simulink model "blockDiagramTask7"  (R2025a)
settings: Solver=VariableStepAuto  StartTime=0.0  StopTime=3.6  RelTol=1e-3
InitFcn:
  | run motor_specs.m
model workspace: external: MATLAB File motor_specs.m (data not in the file)
values from neighbouring files (symbols this model uses):
  A6 = [ 0, 0, 1, 0 ... (first row only)    [ssAndTF.m]
  B6 = [0, 0, K_M/(J_gm*R), 0]'    [ssAndTF.m]
  b_m = C_V / rpm_to_rs    (= 1.05042262441e-05)    [motor_specs.m]
  C6 = eye(4)    [ssAndTF.m]
  J = 6.3E-6    (= 6.3e-06)    [motor_specs.m]
  K_E = 0.006741 / rpm_to_rs    (= 0.0643718082829)    [motor_specs.m]
  K_M = 0.0644    [motor_specs.m]
  R = 3.23    [motor_specs.m]
  U_N = 36    [motor_specs.m]
undefined symbols (not defined in the file or in its folder): sigbuilder_block
libraries: fl_lib x4, nesl_utility x3, ee_lib x1, slpidlib x1
settings Model: Creator=josef  LastModifiedBy=josef

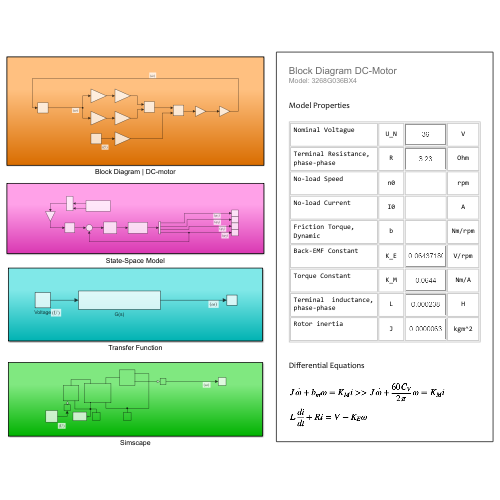
[thumbnail: Simulink's stored preview of the top-level diagram]
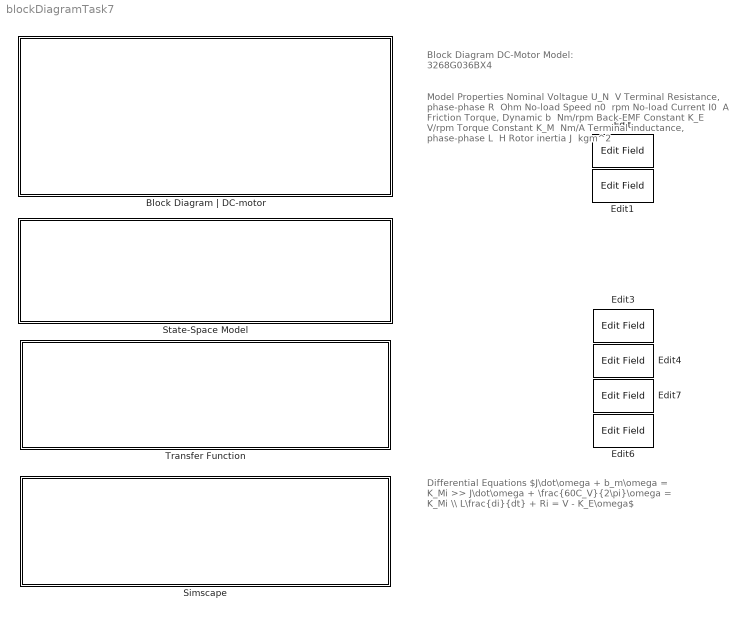
== system blockDiagramTask7 ==
  note: Differential Equations
      |
      | $J\dot\omega + b_m\omega = K_Mi >> J\dot\omega + \frac{60C_V}{2\pi}\omega = K_Mi \\ L\frac{di}{dt} + Ri = V - K_E\omega$
  note: Model Properties
      |
      | Nominal Voltague
      |
      | U_N
      | ​
      | V
      |
      | Terminal Resistance,
      | phase-phase
      | R
      | ​
      | Ohm
      |
      | No-load Speed
      |
      | n0
      | ​
      | rpm
      |
      | No-load Current
      |
      | I0
      | ​
      | A
      |
      | Friction Torque,
      | Dynamic
      | b
      | ​
      | Nm/rpm
      |
      | Back-EMF Constant
      |
      | K_E
      | ​
      | V/rpm
      |
      | Torque Constant
      |
      | K_M
      | ​
      | Nm/A
      |
      | Terminal inductance,
      | phase-phase
      | L
      | ​
      | H
      |
      | Rotor inertia
      |
      | J
      | ​
      | kgm^2
  note: Block Diagram DC-Motor
      | Model: 3268G036BX4
  Block Diagram | DC-motor : Subsystem
  Edit{,1,3..4,6..7} (6 alike) : EditField  LabelPosition=Hide  ShowInitialText=on  Alignment=Center  Opacity=0
  Simscape : Subsystem
  State-Space Model : Subsystem
  Transfer Function : Subsystem

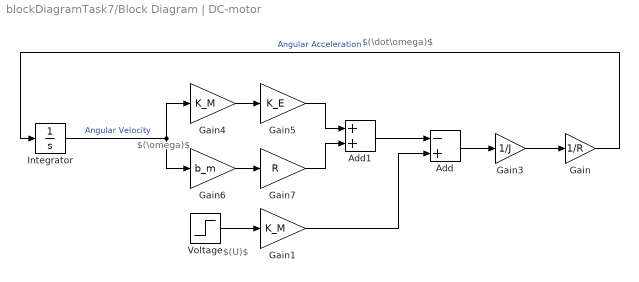
== system blockDiagramTask7/Block Diagram | DC-motor ==
  note: $(\omega)$
  note: $(\dot\omega)$
  note: $(U)$
  Add : Sum  Inputs=-+
  Add1 : Sum
  Gain : Gain  Gain=1/R
  Gain1 : Gain  Gain=K_M
  Gain3 : Gain  Gain=1/J
  Gain4 : Gain  Gain=K_M
  Gain5 : Gain  Gain=K_E
  Gain6 : Gain  Gain=b_m
  Gain7 : Gain  Gain=R
  Integrator : Integrator
  Voltage : Step  Time=0  After=U_N  SampleTime=0
  wires:
  Add1/1 -> Add/1
  Gain4/1 -> Gain5/1
  Gain1/1 -> Add/2
  Gain3/1 -> Gain/1
  Gain5/1 -> Add1/1
  Integrator/1 -> Gain6/1, Gain4/1  "Angular Velocity"
  Gain6/1 -> Gain7/1
  Voltage/1 -> Gain1/1
  Gain/1 -> Integrator/1  "Angular Acceleration"
  Gain7/1 -> Add1/2
  Add/1 -> Gain3/1

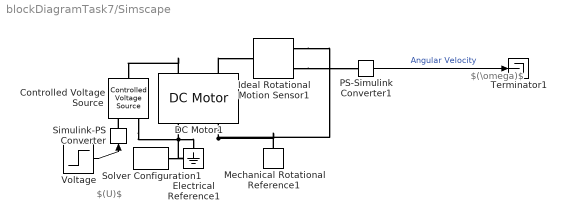
== system blockDiagramTask7/Simscape ==
  note: $(\omega)$
  note: $(U)$
  Controlled Voltage Source : fl_lib/Electrical/Electrical Sources/Controlled Voltage Source
  DC Motor1 : ee_lib/Electromechanical/Brushed Motors/DC Motor  field_option=ee.enum.field_option.pm  Rf=100 Ohm  Lf=1 H  Laf=0.15 H  If0=0 A  parameterization=ee.enum.dcparam_option.circuit_param  Ra=R Ohm  La=0 H  emf_or_torque=ee.enum.emf_or_torque.kv  Kv=K_E V*s/rad  Ki=6.876e-4 N*m/A  T_stall=0.24e-3 N*m  w_max=19100 rpm  w_rated=15000 rpm  P_rated=0.08 W  V_rated=1.5 V  lam_param=ee.enum.lam_param.damping  i_noload=0 A  V_i_noload=1.5 V  J=J kg*m^2  lam=b_m N*m*s/rad  speed0=0 rpm  alpha=3.93e-3 1/K  Tmeas=25 degC  thermal_mass=100 J/K  initial_temperature=25 degC
  Electrical Reference1 : fl_lib/Electrical/Electrical Elements/Electrical Reference
  Ideal Rotational Motion Sensor1 : fl_lib/Mechanical/Mechanical Sensors/Ideal Rotational Motion Sensor  reference=foundation.enum.MeasurementReference.difference  acceleration_port=false  velocity_port=true  position_port=false  wrap_angle=false  offset=0 rad
      settings: InternalSimscapePortConfiguration="{\"Bottom\":[],\"Left\":[{\"id\":\"R\",\"label\":\"R\",\"type\":\"foundation.mechanical.rotational.rotational\"}],\"Right\":[{\"id\":\"C\",\"label\":\"C\",\"type\":\"foundation.mechanical.rotational.rotational\"},{\"id\":\"W\",\"label\":\"W\",\"type\":\"output\"}],\"Top\":[]}"
  Mechanical Rotational Reference1 : fl_lib/Mechanical/Rotational Elements/Mechanical Rotational Reference
  PS-Simulink Converter1 : nesl_utility/PS-Simulink Converter  PhysicalDomain=network_engine_domain  SubClassName=ps_output  LeftPortType=input  RightPortType=output  PseudoPeriodic=off  Frequencies=[]  VectorFormat=inherit  Unit=inherit  AffineConversion=off
  Simulink-PS Converter : nesl_utility/Simulink-PS Converter  PhysicalDomain=network_engine_domain  SubClassName=ps_input  LeftPortType=input  RightPortType=output  PseudoPeriodic=off  Frequencies=[]  NoiseDistribution=none  NoiseParameters=[]  Unit=1  AffineConversion=off  FilteringAndDerivatives=provide  SimscapeFilterOrder=1  InputFilterTimeConstant=0.001  UdotUserProvided=0
  Solver Configuration1 : nesl_utility/Solver Configuration  PhysicalDomain=network_engine_domain  SubClassName=solver  LeftPortType=input  RightPortType=generic  Tones=[]  Harmonics=[]  SimulateNoise=off  Profile=off  UseLocalSampling=off  EnableSwitchedLinearOptims=on  FrequencyDomain=off  UseCCode=off  RelTol=0.001  AbsTol=0.001  MinStep=1e-09  ToWorkspace=off  RevertToSquareIcSolve=off  NumHomotopyIterations=100  PhasorMode=off  PhasorModeNumHarmonics=1  ConsistencySolver=NEWTON_XTOL_AFTER_FTOL  IndexReductionMethod=DerivativeReplacement  DoDC=off  ResidualTolerance=1e-09  ConsistencyTolSource=GLOBAL  ConsistencyAbsTol=0.001  ConsistencyRelTol=0.001  ConsistencyTolFactor=0.001  UseLocalSolver=off  LocalSolverChoice=NE_BACKWARD_EULER_ADVANCER  ResolveIndetEquations=on  FunctionEvalNumThread=1  LocalSolverSampleTime=0.001  DoFixedCost=off  MaxNonlinIter=3  MaxModeIter=2  ComputeImpulses=off  ImpulseIterations=2  LinearAlgebra=auto  LinearAlgebraNumThread=0  EquationFormulation=NE_TIME_EF  DelaysMemoryBudget=1024  AutomaticFiltering=on  FilteringTimeConstant=0.001  PartitionStorageMethod=AS_NEEDED  PartitionMemoryBudget=1024  PartitionMethod=ROBUST  MultibodyUseLocalSolver=off  MultibodyLocalSolverChoice=ODE1  MultibodyLocalSolverSampleTime=0.001
  Terminator1 : Terminator
  Voltage : Step  Time=0.1  After=U_N  SampleTime=0
  wires:
  PS-Simulink Converter1/1 -> Terminator1/1  "Angular Velocity"
  Voltage/1 -> Simulink-PS Converter/1
  connections:
  Solver Configuration1/RConn1 -- Controlled Voltage Source/RConn2 -- Electrical Reference1/LConn1 -- DC Motor1/RConn1
  DC Motor1/RConn2 -- Ideal Rotational Motion Sensor1/RConn1 -- Mechanical Rotational Reference1/LConn1
  Ideal Rotational Motion Sensor1/RConn2 -- PS-Simulink Converter1/LConn1
  Simulink-PS Converter/RConn1 -- Controlled Voltage Source/RConn1
  DC Motor1/LConn1 -- Controlled Voltage Source/LConn1
  DC Motor1/LConn2 -- Ideal Rotational Motion Sensor1/LConn1

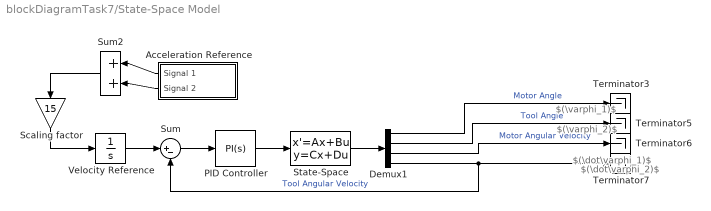
== system blockDiagramTask7/State-Space Model ==
  note: $(\varphi_1)$
  note: $(\varphi_2)$
  note: $(\dot\varphi_2)$
  note: $(\dot\varphi_1)$
  Acceleration Reference : Subsystem  Tag=STV Subsys  LoadFcn=sigbuilder_block('load');  StartFcn=sigbuilder_block('start');  StopFcn=sigbuilder_block('stop');  ClipboardFcn=sigbuilder_block('clipboard');  mask(Sigbuilder block){tuvar=[0:10]}
      mask help: Sigbuilder GUI
      mask init:
      | if ~strcmp(get_param(bdroot(gcbh),'SimulationStatus'),'stopped') tuvar = sigbuilder_block('maskInit'); end
      settings: CopyFcn=sigbuilder_block('copy');  DeleteFcn=sigbuilder_block('delete');  ModelCloseFcn=sigbuilder_block('modelClose');  PreSaveFcn=sigbuilder_block('preSave');  PauseFcn=sigbuilder_block('pause')  ContinueFcn=sigbuilder_block('continue')  NameChangeFcn=sigbuilder_block('namechange');  OpenFcn=sigbuilder_block('open',[316.5 171.75 805.5 485.25 ]);  CloseFcn=sigbuilder_block('close');
      mask Display: plot(0, 0, 100, 100,[2, 2, 32, 32, 2], [68, 8, 8, 68, 68],[32, 2], [38, 38], [32, 19, 2],[53, 60, 44], [32, 17, 17, 2],[16, 16, 31, 31]);txt = getActiveGroup(gcbh);text(2, 100, txt,'verticalAlignment', 'top');
  Demux1 : Demux
  PID Controller : slpidlib/PID Controller  Controller=PI  Form=Parallel  TimeDomain=Continuous-time  UseExternalTs=off  SampleTime=-1  IntegratorMethod=Forward Euler  FilterMethod=Forward Euler  ControllerParametersSource=internal  P=1  I=1  UseKiTs=off  D=0  UseExternalDerivativeSource=off  N=100  UseFilter=on  TunerSelectOption=Transfer Function Based (PID Tuner App)  InitialConditionSource=internal  InitialConditionForIntegrator=0  InitialConditionForFilter=0  DifferentiatorICPrevScaledInput=0  ExternalReset=none  TrackingMode=off  Kt=1  LimitOutput=off  SatLimitsSource=internal  UpperSaturationLimit=inf  LowerSaturationLimit=-inf  LinearizeAsGain=on  AntiWindupMode=none  Kb=1  LimitIntegrator=off  UpperIntegratorSaturationLimit=inf  LowerIntegratorSaturationLimit=-inf  POutMin=[]  POutMax=[]  IOutMin=[]  IOutMax=[]  DOutMin=[]  DOutMax=[]  NOutMin=[]  NOutMax=[]  SumOutMin=[]  SumOutMax=[]  SaturationOutMin=[]  SaturationOutMax=[]  PParamMin=[]  PParamMax=[]  IParamMin=[]  IParamMax=[]  DParamMin=[]  DParamMax=[]  NParamMin=[]  NParamMax=[]  KbParamMin=[]  KbParamMax=[]  KtParamMin=[]  KtParamMax=[]  KbOutMin=[]  KbOutMax=[]  KtOutMin=[]  KtOutMax=[]  IntegratorOutMin=[]  IntegratorOutMax=[]  FilterOutMin=[]  FilterOutMax=[]  SumI1OutMin=[]  SumI1OutMax=[]  SumI2OutMin=[]  SumI2OutMax=[]  SumI3OutMin=[]  SumI3OutMax=[]  SumI4OutMin=[]  SumI4OutMax=[]  SumDOutMin=[]  SumDOutMax=[]  DifferentiatorOutMin=[]  DifferentiatorOutMax=[]  FilterDiffOutCoefMin=[]  FilterDiffOutCoefMax=[]  ReciprocalOutMin=[]  ReciprocalOutMax=[]  SumDenOutMin=[]  SumDenOutMax=[]  SumNumOutMin=[]  SumNumOutMax=[]  DivideOutMin=[]  DivideOutMax=[]  UdiffTsProdOutMin=[]  UdiffTsProdOutMax=[]  NTsProdOutMin=[]  NTsProdOutMax=[]  UintegralTsProdOutMin=[]  UintegralTsProdOutMax=[]  UngainTsProdOutMin=[]  UngainTsProdOutMax=[]  ClampingZeroOutDataTypeStr=Inherit: Inherit via back propagation  ClampingZeroOutMin=[]  ClampingZeroOutMax=[]  FilterDenConstantOutDataTypeStr=Inherit: Inherit via back propagation  FilterDenConstantOutMin=[]  FilterDenConstantOutMax=[]  PCopyOutDataTypeStr=Inherit: Inherit via back propagation  PCopyOutMin=[]  PCopyOutMax=[]  NCopyOutDataTypeStr=Inherit: Inherit via back propagation  NCopyOutMin=[]  NCopyOutMax=[]  IntegratorContinuousStateAttributes=''  IntegratorStateMustResolveToSignalObject=off  IntegratorRTWStateStorageClass=Auto  FilterContinuousStateAttributes=''  FilterStateMustResolveToSignalObject=off  FilterRTWStateStorageClass=Auto  ParallelPVariant=InternalParameters  IdealPVariant=Disabled  IVariant=InternalParameters  DVariant=Disabled  IntegratorVariant=Continuous  SatVariant=Disabled  AWVariant=Passthrough  PCopyVariant=Disabled  TRVariant=Disabled  FdbkBlocksVariant=Forward  IdealPFdbkVariant=Disabled  SatFdbkVariant=Disabled  DerivativeFilterVariant=Disabled  NVariant=Disabled  NCopyVariant=Disabled_SignalSpec  FilterICVariant=Disabled  IntegratorICVariant=InternalICs  ExternalResetVariant=Disabled  TRSumVariant=Passthrough  SumFdbkVariant=Disabled  SumVariant=Sum_PI  TsampFilterVariant=InternalTs  TsampNgainVariant=Passthrough  TsampIntegralVariant=Disabled_SignalSpec  ExternalSaturationOutDataTypeStr=Inherit: Same as second input  DerivativeSourceVariant=Disabled  PreIntVariant=InternalPreInt
  Scaling factor : Gain  Gain=15
  State-Space : StateSpace  A=A6  B=B6  C=C6  D=[0;0;0;0]  InitialCondition=0
  Sum : Sum  Inputs=|+-
  Sum2 : Sum  Inputs=|++
  Terminator{3,5..7} (4 alike) : Terminator
  Velocity Reference : Integrator
  wires:
  Scaling factor/1 -> Velocity Reference/1
  PID Controller/1 -> State-Space/1
  Sum/1 -> PID Controller/1
  Velocity Reference/1 -> Sum/1
  Sum2/1 -> Scaling factor/1
  Acceleration Reference/2(Signal 2) -> Sum2/2
  Acceleration Reference/1(Signal 1) -> Sum2/1
  Demux1/1 -> Terminator3/1  "Motor Angle"
  Demux1/2 -> Terminator5/1  "Tool Angle"
  Demux1/3 -> Terminator6/1  "Motor Angular Velocity"
  Demux1/4 -> Sum/2, Terminator7/1  "Tool Angular Velocity"
  State-Space/1 -> Demux1/1

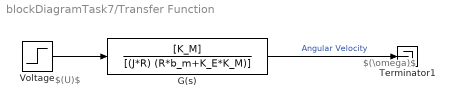
== system blockDiagramTask7/Transfer Function ==
  note: $(\omega)$
  note: $(U)$
  G(s) : TransferFcn  Numerator=[K_M]  Denominator=[(J*R) (R*b_m+K_E*K_M)]
  Terminator1 : Terminator
  Voltage : Step  Time=0.1  After=U_N  SampleTime=0
  wires:
  G(s)/1 -> Terminator1/1  "Angular Velocity"
  Voltage/1 -> G(s)/1

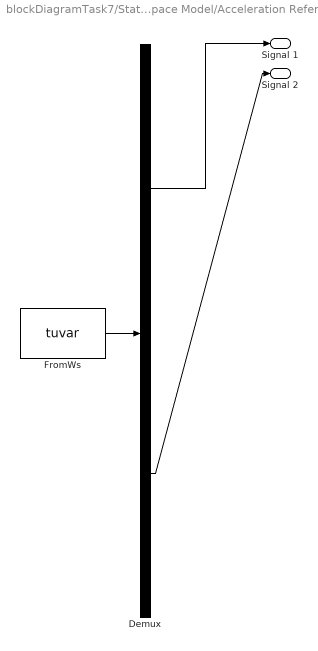
== system blockDiagramTask7/State-Space Model/Acceleration Reference ==
  Demux : Demux  Tag=STV Demux  Outputs=2
      settings: DisplayOption=none
  FromWs : FromWorkspace  Tag=STV FromWs  VariableName=tuvar
      SigBuilderData=|
      | common.afterFinalStr = 'Extrapolate'
      | common.sampleTime = 0
      | dataSet.timeRange = [0 10]
      | dataSet.name = 'Group 1'
      | sbobj.Groups.Name = 'Group 1'
      | sbobj.Groups.Signals(1).Name = 'Signal 1'
      | sbobj.Groups.Signals(1).XData = [0 0.2 0.2 10]
      | sbobj.Groups.Signals(1).YData = [1 1 0 0]
      | sbobj.Groups.Signals(2).Name = 'Signal 2'
      | sbobj.Groups.Signals(2).XData = [0 2.8 2.8 3 3 10]
      | sbobj.Groups.Signals(2).YData = [0 0 -1 -1 0 0]
  Signal 1 : Outport  Tag=STV Outport
  Signal 2 : Outport  Tag=STV Outport  Port=2
  wires:
  Demux/1 -> Signal 1/1
  FromWs/1 -> Demux/1
  Demux/2 -> Signal 2/1
